simulink model "clotoid"  (R2020b)
settings: Solver=FixedStepAuto  StartTime=0.0  StopTime=60*60  FixedStep=1  RelTol=1e-3
undefined symbols (not defined in the file or in its folder): sigbuilder_block
libraries: aerolibactuator x2
settings Model: Creator=Rafael.Casado  LastModifiedBy=Rafael.Casado

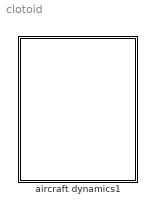
== system clotoid ==
  aircraft dynamics1 : Subsystem
      mask Display:
      | patch([50 -50 -50 50], [40 40 -60 -60], [1 1 1])
      | 
      | patch([8 -8 -8 8], [6 6 -6 -6], [0.7 0.7 0.7])
      | 
      | patch([ 8  8  28  28], [0 -2 2 4], [0.5 0.5 0.5])
      | patch([-8 -8 -28 -28], [0 -2 2 4], [0.5 0.5 0.5])
      | 
      | patch([1 0 -1], [6 18 6], [0.5 0.5 0.5])

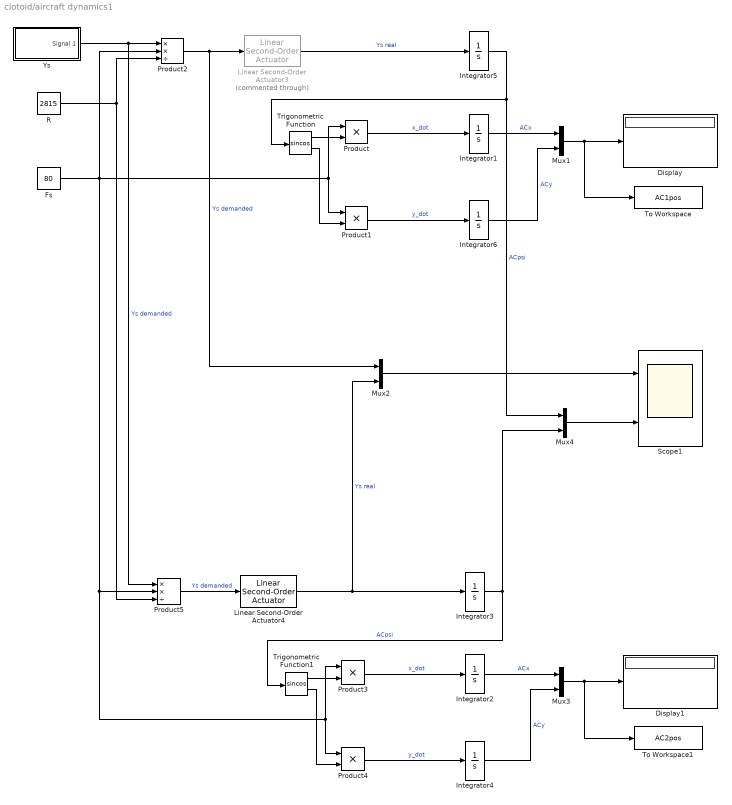
== system clotoid/aircraft dynamics1 ==
  Display : Display
      settings: Decimation=2
  Display1 : Display
      settings: Decimation=2
  Fs : Constant  Value=80
  Integrator{1..6} (6 alike) : Integrator
  Linear Second-Order Actuator3 : aerolibactuator/Linear Second-Order Actuator  Commented=through  wn_fin=1  z_fin=1  fin_act_0=0  fin_act_vel=0
      settings: SourceProductBaseCode=AE
  Linear Second-Order Actuator4 : aerolibactuator/Linear Second-Order Actuator  wn_fin=1  z_fin=1  fin_act_0=0  fin_act_vel=0
      settings: SourceProductBaseCode=AE
  Mux{1..4} (4 alike) : Mux  Inputs=2
  Product{,1,3..4} (4 alike) : Product
  Product2 : Product  Inputs=**/
  Product5 : Product  Inputs=**/
  R : Constant  Value=2815
  Scope1 : Scope  NumInputPorts=2
  To Workspace : ToWorkspace  VariableName=AC1pos  SaveFormat=Timeseries  SampleTime=-1
  To Workspace1 : ToWorkspace  VariableName=AC2pos  SaveFormat=Timeseries  SampleTime=-1
  Trigonometric Function : Trigonometry  Operator=sincos
  Trigonometric Function1 : Trigonometry  Operator=sincos
  Ys : Subsystem  Tag=STV Subsys  LoadFcn=sigbuilder_block('load');  StartFcn=sigbuilder_block('start');  StopFcn=sigbuilder_block('stop');  ClipboardFcn=sigbuilder_block('clipboard');  mask(Sigbuilder block){tuvar=[0:10]}
      mask help: Simulink:masks:SigbuilderBlock_MD
      mask init:
      | if ~strcmp(get_param(bdroot(gcbh),'SimulationStatus'),'stopped') tuvar = sigbuilder_block('maskInit'); end
      settings: CopyFcn=sigbuilder_block('copy');  DeleteFcn=sigbuilder_block('delete');  ModelCloseFcn=sigbuilder_block('modelClose');  PreSaveFcn=sigbuilder_block('preSave');  PauseFcn=sigbuilder_block('pause');  ContinueFcn=sigbuilder_block('continue');  NameChangeFcn=sigbuilder_block('namechange');  OpenFcn=sigbuilder_block('open',[924.6 14.4 1128.6 227.4 ]);  CloseFcn=sigbuilder_block('close');
      mask Display: plot(0, 0, 100, 100,[2, 2, 32, 32, 2], [68, 8, 8, 68, 68],[32, 2], [38, 38], [32, 19, 2],[53, 60, 44], [32, 17, 17, 2],[16, 16, 31, 31]);txt = getActiveGroup(gcbh);text(2, 100, txt,'verticalAlignment', 'top');
  wires:
  Integrator5/1 -> Mux4/1, Trigonometric Function/1  "ACpsi"
  Integrator6/1 -> Mux1/2  "ACy"
  Product2/1 -> Mux2/1, Linear Second-Order Actuator3/1  "Ys demanded"
  Trigonometric Function/2 -> Product1/2
  Product/1 -> Integrator1/1  "x_dot"
  Product1/1 -> Integrator6/1  "y_dot"
  Trigonometric Function/1 -> Product/2
  Linear Second-Order Actuator3/1 -> Integrator5/1  "Ys real"
  Mux1/1 -> To Workspace/1, Display/1
  Integrator1/1 -> Mux1/1  "ACx"
  Ys/1(Signal 1) -> Product5/1, Product2/1  "Ys demanded"
  R/1 -> Product5/3, Product2/3
  Mux2/1 -> Scope1/1
  Trigonometric Function1/1 -> Product3/2
  Product4/1 -> Integrator4/1  "y_dot"
  Integrator4/1 -> Mux3/2  "ACy"
  Fs/1 -> Product/1, Product1/1, Product3/1, Product4/1, Product5/2, Product2/2
  Product3/1 -> Integrator2/1  "x_dot"
  Trigonometric Function1/2 -> Product4/2
  Mux3/1 -> To Workspace1/1, Display1/1
  Integrator3/1 -> Trigonometric Function1/1, Mux4/2  "ACpsi"
  Linear Second-Order Actuator4/1 -> Integrator3/1, Mux2/2  "Ys real"
  Integrator2/1 -> Mux3/1  "ACx"
  Product5/1 -> Linear Second-Order Actuator4/1  "Ys demanded"
  Mux4/1 -> Scope1/2

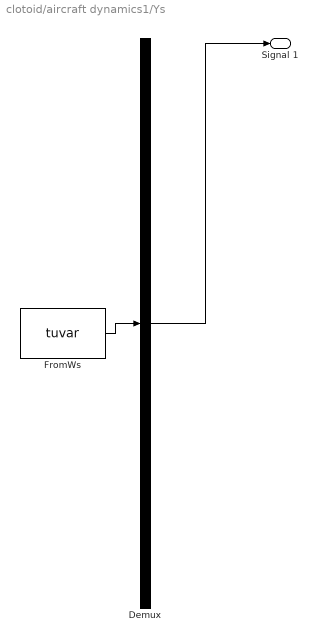
== system clotoid/aircraft dynamics1/Ys ==
  Demux : Demux  Tag=STV Demux  Outputs=1
      settings: DisplayOption=none
  FromWs : FromWorkspace  Tag=STV FromWs  VariableName=tuvar
      SigBuilderData=|
      | common.afterFinalStr = 'Extrapolate'
      | common.sampleTime = 0
      | dataSet.timeRange = [0 3600]
      | dataSet.name = 'Group 1'
      | sbobj.Groups.Name = 'Group 1'
      | sbobj.Groups.Signals.Name = 'Signal 1'
      | sbobj.Groups.Signals.XData = [0 693 693 770 770 2071 2071 2164 2164 3600]
      | sbobj.Groups.Signals.YData = [0 0 1 1 0 0 1 1 0 0]
      | sbobj.Groups.TimeRange = [0 3600]
  Signal 1 : Outport  Tag=STV Outport
  wires:
  Demux/1 -> Signal 1/1
  FromWs/1 -> Demux/1
